simulink model "gm_sampleModel1758_sub_sub_sub"  (R2023a)
settings: Solver=VariableStepAuto  StartTime=0.0  StopTime=10.0  RelTol=1e-3
libraries: hdlsllib x4, simulink x1
settings Model: Creator=user1  LastModifiedBy=user1
settings OptimizationCC: BlockReduction=off  ConditionallyExecuteInputs=off
settings DebuggingCC: InheritedTsInSrcMsg=none

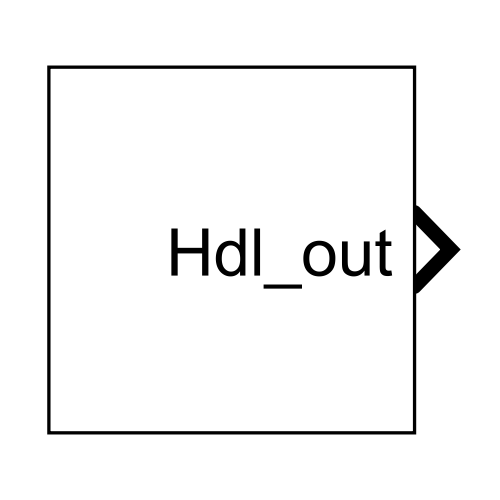
[thumbnail: Simulink's stored preview of the top-level diagram]
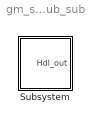
== system gm_sampleModel1758_sub_sub_sub ==
  Subsystem : Subsystem

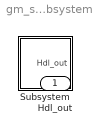
== system gm_sampleModel1758_sub_sub_sub/Subsystem ==
  Subsystem : Subsystem
  Hdl_out : Outport  OutDataTypeStr=uint8

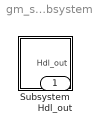
== system gm_sampleModel1758_sub_sub_sub/Subsystem/Subsystem ==
  Subsystem : Subsystem
  Hdl_out : Outport  OutDataTypeStr=uint8

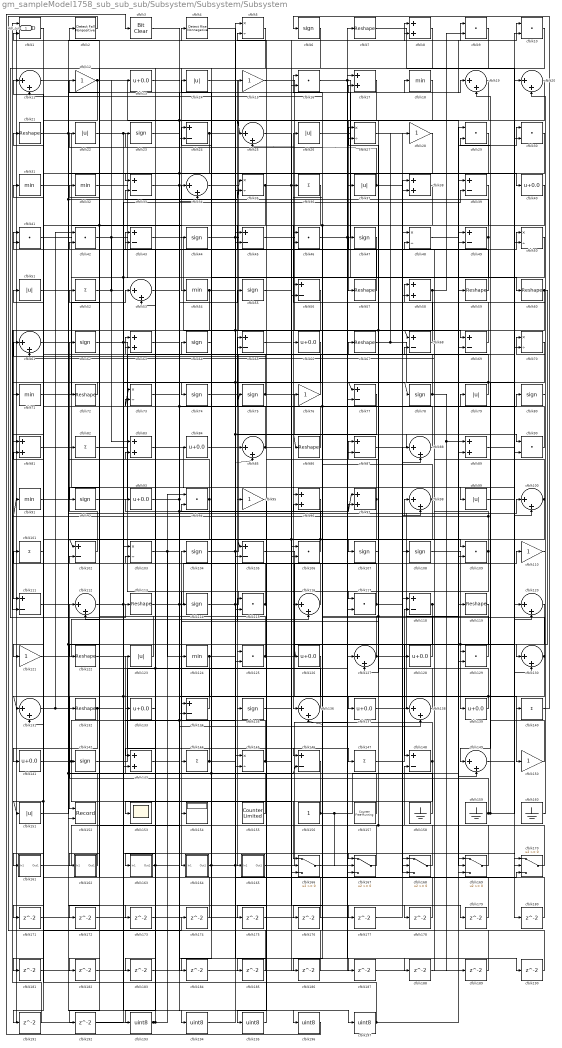
== system gm_sampleModel1758_sub_sub_sub/Subsystem/Subsystem/Subsystem ==
  cfblk1 : Logic  AllPortsSameDT=off  OutDataTypeStr=boolean
  cfblk{9..10,16,29..30,41..42,46,90,94,106,109,115,117,125,129} (16 alike) : DotProduct  OutDataTypeStr=uint8
  cfblk{11,19..20,25,34,53,61,85,88,98,100,112,116,120,127,130..131,136,138,149} (20 alike) : Sum  Inputs=|++  OutDataTypeStr=uint8
  cfblk{36,52,82,101,140,144,147} (7 alike) : Sum  Inputs=+  OutDataTypeStr=uint8
  cfblk{24,33,39,43,45,49,56,65,68..69,77,87,102,105,111,118,134,146,148} (19 alike) : Sum  Inputs=+-  OutDataTypeStr=uint8
  cfblk{5,27,35,48,50,70,73,103,145} (9 alike) : Product  Inputs=*/  OutDataTypeStr=uint8  RndMeth=Zero  SaturateOnIntegerOverflow=on
  cfblk{6,23,44,47,55,62,64,74..75,78,80,92,104,107..108,114,135,142} (18 alike) : Signum
  cfblk{12,15,28,76,95,110,121,150} (8 alike) : Gain  OutDataTypeStr=uint8
  cfblk{7,21,57,59..60,67,72,86,113,119,122,132} (12 alike) : Reshape
  cfblk{14,22,26,37,51,79,99,123,151} (9 alike) : Abs  OutDataTypeStr=uint8  SaturateOnIntegerOverflow=off
  cfblk{18,31..32,54,71,91,124} (7 alike) : MinMax  OutDataTypeStr=uint8
  cfblk{13,40,66,84,93,126,128,133,137,139,141} (11 alike) : Bias  Bias=0.0  SaturateOnIntegerOverflow=off
  cfblk{8,17,38,58,63,81,83,89,96..97,143} (11 alike) : Sum  OutDataTypeStr=uint8
  cfblk152 : Record  FileSettingsInternal="{\"entries\":[{\"content\":{\"excelSettings\":{\"content\":{},\"type\":\"Streamout.ExcelSettings\"}},\"type\":\"Streamout.FileSettingStorage\",\"uuid\":\"\"}],\"packageUris\":[\"http:\\/\\/schema.mathworks.com\\/mf0\\/streamout_blocks\\/R2020a\"],\"version\":\"1.0\"}"  Layout=[1 1]  SignalsInternal="{\"entries\":[{\"content\":{\"signals\":[{\"content\":{\"blockPath\":[],\"dimensions\":[1],\"domain\":\"\",\"lineColor\":\"#a2142f\",\"plots\":[1],\"port\":1,\"signalID\":40096,\"signalName\":\"cfblk126\"},\"type\":\"RecordBlkView.Signal\",\"uuid\":\"\"},{\"content\":{\"blockPath\":[],\"dimensions\":[1],\"domain\":\"\",\"lineColor\":\"#139fff\",\"plots\":[1],\"port\":2,\"signalID\":40099,\"signalName\":\"cfblk94\"},\"type\":\"RecordBlkView.Signal\",\"uuid\":\"\"}]},\"type\":\"RecordBlkView.InputSignals\",\"uuid\":\"\"}],\"packageUris\":[\"http:\\/\\/schema.mathworks.com\\/mf0\\/streamout_blocks\\/R2020a\"],\"version\":\"1.0\"}"  VisualizationBindings="{\"xyplotplugin\":{\"info\":[{\"series\":[{\"bindingParametersList\":[{\"parameter\":\"X-Axis\",\"signalID\":40096,\"signalName\":\"cfblk126\"},{\"parameter\":\"Y-Axis\",\"signalID\":40099,\"signalName\":\"cfblk94\"}],\"seriesID\":50755}],\"subplotID\":1}]}}"  CompatibilityTag=XY  st=-1
  cfblk153 : Scope
  cfblk154 : Display
  cfblk155 : hdlsllib/Sources/Counter Limited  uplimit=7  tsamp=-1
  cfblk156 : Constant  OutDataTypeStr=uint8  SampleTime=-1
  cfblk157 : hdlsllib/Sources/Counter Free-Running  NumBits=16  tsamp=-1
  cfblk158 : Ground
  cfblk159 : Ground
  cfblk160 : Ground
  cfblk161 : Subsystem
      settings: LibrarySourceBlock=|
      | hdlsllib/Ports &
      | Subsystems/Subsystem
  cfblk162 : Subsystem
      settings: LibrarySourceBlock=|
      | hdlsllib/Ports &
      | Subsystems/Subsystem
  cfblk163 : Subsystem
      settings: LibrarySourceBlock=|
      | hdlsllib/Ports &
      | Subsystems/Subsystem
  cfblk164 : Subsystem
      settings: LibrarySourceBlock=|
      | hdlsllib/Ports &
      | Subsystems/Subsystem
  cfblk165 : Subsystem
      settings: LibrarySourceBlock=|
      | hdlsllib/Ports &
      | Subsystems/Subsystem
  cfblk{166..170} (5 alike) : Switch  OutDataTypeStr=uint8  SaturateOnIntegerOverflow=off  InputSameDT=off
  cfblk{171..192} (22 alike) : Delay  SampleTime=1
  cfblk{193..197} (5 alike) : DataTypeConversion  OutDataTypeStr=uint8  SaturateOnIntegerOverflow=off  RndMeth=Floor
  cfblk2 : hdlsllib/Logic and Bit Operations/Detect Fall Nonpositive  vinit=0  OutDataTypeStr=uint8
  cfblk3 : simulink/Logic and Bit Operations/Bit Clear  iBit=0
      settings: LibrarySourceBlock=|
      | hdlsllib/Logic and Bit
      | Operations/Bit Clear
  cfblk4 : hdlsllib/Logic and Bit Operations/Detect Rise Nonnegative  vinit=0  OutDataTypeStr=uint8
  Hdl_out : Outport  OutDataTypeStr=uint8
  wires:
  cfblk197/1 -> cfblk89/2, cfblk51/1
  cfblk196/1 -> cfblk3/1
  cfblk195/1 -> cfblk5/2
  cfblk175/1 -> cfblk195/1
  cfblk194/1 -> cfblk5/1
  cfblk193/1 -> cfblk73/2, cfblk94/1, Hdl_out/1
  cfblk192/1 -> cfblk103/1
  cfblk191/1 -> cfblk1/1
  cfblk190/1 -> cfblk96/2
  cfblk189/1 -> cfblk94/2
  cfblk188/1 -> cfblk98/1
  cfblk187/1 -> cfblk49/1
  cfblk186/1 -> cfblk41/2
  cfblk120/1 -> cfblk186/1
  cfblk185/1 -> cfblk45/1
  cfblk184/1 -> cfblk16/2
  cfblk64/1 -> cfblk184/1
  cfblk183/1 -> cfblk169/3
  cfblk182/1 -> cfblk127/1
  cfblk30/1 -> cfblk182/1
  cfblk181/1 -> cfblk34/2
  cfblk180/1 -> cfblk106/1
  cfblk149/1 -> cfblk180/1
  cfblk179/1 -> cfblk145/1
  cfblk51/1 -> cfblk179/1
  cfblk178/1 -> cfblk17/1
  cfblk166/1 -> cfblk178/1
  cfblk177/1 -> cfblk88/1
  cfblk65/1 -> cfblk177/1
  cfblk176/1 -> cfblk81/2
  cfblk95/1 -> cfblk175/1
  cfblk174/1 -> cfblk102/2
  cfblk2/1 -> cfblk174/1
  cfblk173/1 -> cfblk53/2
  cfblk172/1 -> cfblk168/2
  cfblk171/1 -> cfblk168/1
  cfblk101/1 -> cfblk171/1
  cfblk80/1 -> cfblk20/2
  cfblk159/1 -> cfblk30/2, cfblk29/2, cfblk142/1
  cfblk141/1 -> cfblk45/2, cfblk24/2, cfblk166/2
  cfblk115/1 -> cfblk42/2, cfblk185/1
  cfblk73/1 -> cfblk99/1
  cfblk37/1 -> cfblk168/3, cfblk25/2
  cfblk34/1 -> cfblk119/1
  cfblk82/1 -> cfblk49/2
  cfblk139/1 -> cfblk131/1, cfblk114/1
  cfblk130/1 -> cfblk11/2, cfblk172/1
  cfblk100/1 -> cfblk46/2, cfblk176/1
  cfblk48/1 -> cfblk30/1
  cfblk23/1 -> cfblk17/2
  cfblk45/1 -> cfblk129/2
  cfblk89/1 -> cfblk70/2
  cfblk69/1 -> cfblk47/1
  cfblk123/1 -> cfblk1/2
  cfblk11/1 -> cfblk40/1
  cfblk163/1(Out1) -> cfblk138/1, cfblk43/2
  cfblk66/1 -> cfblk161/1(In1)
  cfblk74/1 -> cfblk29/1
  cfblk162/1(Out1) -> cfblk132/1
  cfblk116/1 -> cfblk31/1
  cfblk53/1 -> cfblk109/1
  cfblk150/1 -> cfblk19/2
  cfblk32/1 -> cfblk56/2
  cfblk55/1 -> cfblk8/2
  cfblk91/1 -> cfblk8/1
  cfblk1/1 -> cfblk81/1
  cfblk160/1 -> cfblk70/1
  cfblk170/1 -> cfblk148/2
  cfblk132/1 -> cfblk151/1, cfblk181/1, cfblk196/1
  cfblk86/1 -> cfblk52/1
  cfblk20/1 -> cfblk127/2
  cfblk148/1 -> cfblk101/1, cfblk154/1
  cfblk42/1 -> cfblk134/2, cfblk83/1
  cfblk85/1 -> cfblk65/2, cfblk128/1
  cfblk17/1 -> cfblk145/2
  cfblk107/1 -> cfblk27/1
  cfblk118/1 -> cfblk148/1, cfblk68/2
  cfblk24/1 -> cfblk115/2, cfblk33/1
  cfblk129/1 -> cfblk23/1, cfblk87/1
  cfblk138/1 -> cfblk115/1
  cfblk9/1 -> cfblk162/1(In1)
  cfblk78/1 -> cfblk89/1, cfblk189/1, cfblk43/1
  cfblk7/1 -> cfblk90/2
  cfblk142/1 -> cfblk79/1
  cfblk96/1 -> cfblk106/2, cfblk105/1
  cfblk164/1(Out1) -> cfblk170/3, cfblk97/2, cfblk14/1
  cfblk92/1 -> cfblk10/2
  cfblk99/1 -> cfblk50/2
  cfblk70/1 -> cfblk149/1
  cfblk168/1 -> cfblk16/1, cfblk27/2
  cfblk90/1 -> cfblk48/2
  cfblk50/1 -> cfblk76/1
  cfblk59/1 -> cfblk15/1
  cfblk33/1 -> cfblk167/1, cfblk38/2
  cfblk161/1(Out1) -> cfblk84/1
  cfblk124/1 -> cfblk143/2, cfblk192/1, cfblk167/3
  cfblk109/1 -> cfblk61/2, cfblk91/1, cfblk117/1
  cfblk108/1 -> cfblk129/1
  cfblk58/1 -> cfblk107/1, cfblk183/1, cfblk9/2
  cfblk167/1 -> cfblk12/1
  cfblk26/1 -> cfblk170/1
  cfblk140/1 -> cfblk6/1
  cfblk36/1 -> cfblk92/1
  cfblk49/1 -> cfblk74/1, cfblk33/2
  cfblk57/1 -> cfblk21/1
  cfblk88/1 -> cfblk41/1
  cfblk18/1 -> cfblk112/2
  cfblk29/1 -> cfblk37/1
  cfblk46/1 -> cfblk10/1, cfblk9/1
  cfblk135/1 -> cfblk147/1
  cfblk128/1 -> cfblk46/1
  cfblk158/1 -> cfblk123/1
  cfblk133/1 -> cfblk163/1(In1)
  cfblk151/1 -> cfblk18/1, cfblk146/2
  cfblk28/1 -> cfblk141/1
  cfblk75/1 -> cfblk120/1, cfblk11/1
  cfblk25/1 -> cfblk100/2
  cfblk157/1 -> cfblk24/1, cfblk103/2
  cfblk113/1 -> cfblk85/1, cfblk117/2
  cfblk93/1 -> cfblk19/1, cfblk137/1
  cfblk14/1 -> cfblk88/2
  cfblk52/1 -> cfblk77/2, cfblk13/1
  cfblk117/1 -> cfblk140/1, cfblk32/1
  cfblk126/1 -> cfblk152/1
  cfblk143/1 -> cfblk67/1, cfblk75/1
  cfblk102/1 -> cfblk82/1
  cfblk147/1 -> cfblk118/2
  cfblk4/1 -> cfblk86/1, cfblk166/3, cfblk78/1, cfblk68/1
  cfblk13/1 -> cfblk35/2, cfblk187/1, cfblk25/1
  cfblk136/1 -> cfblk63/1
  cfblk131/1 -> cfblk42/1, cfblk173/1
  cfblk127/1 -> cfblk22/1, cfblk73/1, cfblk69/2
  cfblk35/1 -> cfblk131/2, cfblk122/1, cfblk108/1, cfblk170/2
  cfblk16/1 -> cfblk98/2, cfblk190/1
  cfblk54/1 -> cfblk60/1, cfblk111/2
  cfblk63/1 -> cfblk146/1
  cfblk121/1 -> cfblk116/2
  cfblk84/1 -> cfblk38/1
  cfblk79/1 -> cfblk77/1, cfblk63/2
  cfblk39/1 -> cfblk136/2, cfblk105/2
  cfblk10/1 -> cfblk134/1
  cfblk146/1 -> cfblk166/1
  cfblk5/1 -> cfblk193/1
  cfblk165/1(Out1) -> cfblk7/1
  cfblk83/1 -> cfblk95/1
  cfblk31/1 -> cfblk56/1
  cfblk76/1 -> cfblk65/1
  cfblk12/1 -> cfblk121/1, cfblk149/2
  cfblk106/1 -> cfblk102/1, cfblk93/1
  cfblk114/1 -> cfblk116/1, cfblk110/1
  cfblk112/1 -> cfblk50/1, cfblk130/2
  cfblk169/1 -> cfblk34/1
  cfblk134/1 -> cfblk2/1, cfblk83/2
  cfblk68/1 -> cfblk26/1
  cfblk119/1 -> cfblk139/1, cfblk126/1
  cfblk105/1 -> cfblk150/1
  cfblk61/1 -> cfblk4/1, cfblk35/1
  cfblk94/1 -> cfblk62/1, cfblk152/2
  cfblk103/1 -> cfblk55/1, cfblk97/1, cfblk124/1
  cfblk22/1 -> cfblk169/2, cfblk58/2, cfblk169/1
  cfblk60/1 -> cfblk130/1, cfblk143/1
  cfblk98/1 -> cfblk125/1, cfblk36/1
  cfblk21/1 -> cfblk44/1, cfblk109/2
  cfblk27/1 -> cfblk48/1
  cfblk122/1 -> cfblk144/1
  cfblk125/1 -> cfblk59/1, cfblk72/1
  cfblk3/1 -> cfblk197/1
  cfblk15/1 -> cfblk118/1
  cfblk137/1 -> cfblk20/1
  cfblk156/1 -> cfblk167/2, cfblk39/1, cfblk153/1
  cfblk19/1 -> cfblk57/1
  cfblk41/1 -> cfblk96/1
  cfblk6/1 -> cfblk54/1
  cfblk81/1 -> cfblk125/2, cfblk194/1
  cfblk97/1 -> cfblk61/1, cfblk191/1
  cfblk71/1 -> cfblk53/1
  cfblk110/1 -> cfblk58/1
  cfblk38/1 -> cfblk135/1
  cfblk145/1 -> cfblk104/1, cfblk138/2
  cfblk62/1 -> cfblk164/1(In1), cfblk39/2
  cfblk111/1 -> cfblk100/1
  cfblk40/1 -> cfblk66/1
  cfblk87/1 -> cfblk90/1
  cfblk155/1 -> cfblk112/1
  cfblk77/1 -> cfblk165/1(In1)
  cfblk104/1 -> cfblk80/1, cfblk85/2
  cfblk72/1 -> cfblk71/1
  cfblk144/1 -> cfblk133/1, cfblk188/1
  cfblk8/1 -> cfblk113/1
  cfblk43/1 -> cfblk136/1
  cfblk44/1 -> cfblk69/1, cfblk87/2
  cfblk47/1 -> cfblk64/1
  cfblk67/1 -> cfblk28/1, cfblk120/2
  cfblk56/1 -> cfblk111/1

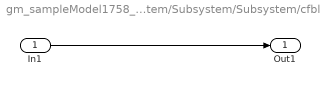
== system gm_sampleModel1758_sub_sub_sub/Subsystem/Subsystem/Subsystem/cfblk161 ==
  In1 : Inport
  Out1 : Outport
  wires:
  In1/1 -> Out1/1

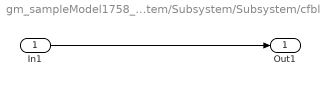
== system gm_sampleModel1758_sub_sub_sub/Subsystem/Subsystem/Subsystem/cfblk162 ==
  In1 : Inport
  Out1 : Outport
  wires:
  In1/1 -> Out1/1

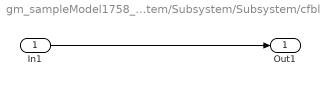
== system gm_sampleModel1758_sub_sub_sub/Subsystem/Subsystem/Subsystem/cfblk163 ==
  In1 : Inport
  Out1 : Outport
  wires:
  In1/1 -> Out1/1

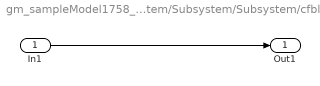
== system gm_sampleModel1758_sub_sub_sub/Subsystem/Subsystem/Subsystem/cfblk164 ==
  In1 : Inport
  Out1 : Outport
  wires:
  In1/1 -> Out1/1

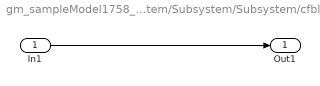
== system gm_sampleModel1758_sub_sub_sub/Subsystem/Subsystem/Subsystem/cfblk165 ==
  In1 : Inport
  Out1 : Outport
  wires:
  In1/1 -> Out1/1
